simulink model "s_aero2_2dof_lqi"  (R2025a)
settings: Solver=ode4  StartTime=0.0  StopTime=30  FixedStep=0.002  RelTol=1e-3
values from neighbouring files (symbols this model uses):
  A = [0 0 1 0 0 0 ... (first row only)    [aero2_2dof_control_lqi.m]
  B = [0 0; 0 0; 0 0; 0 0; Kpp*Dt/Jp Kpy*Dt/Jp; Kyp*Dt/Jy Kyy*Dt/Jy]    [aero2_2dof_control_lqi.m]
  C = [0 0 1 0 0 0; 0 0 0 1 0 0]    [aero2_2dof_control_lqi.m]
  D = zeros(2)    [aero2_2dof_control_lqi.m]
  K = lqr(A, B, Q, R)    [aero2_2dof_control_lqi.m]
libraries: simulink_extras x4, quarc_library x4
settings Model: Creator=MLevis  LastModifiedBy=khanh
settings DataIOCC: ReturnWorkspaceOutputs=off
settings DebuggingCC: UnconnectedInputMsg=warning  UnconnectedOutputMsg=warning  UnconnectedLineMsg=warning
settings ModelReferenceCC: EnableRefExpFcnMdlSchedulingChecks=on
settings RTWCC: GPUComputeCapability=3.5  DLArmComputeVersion=19.05

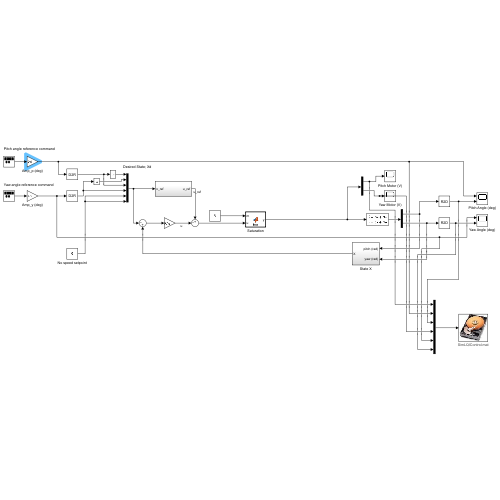
[thumbnail: Simulink's stored preview of the top-level diagram]
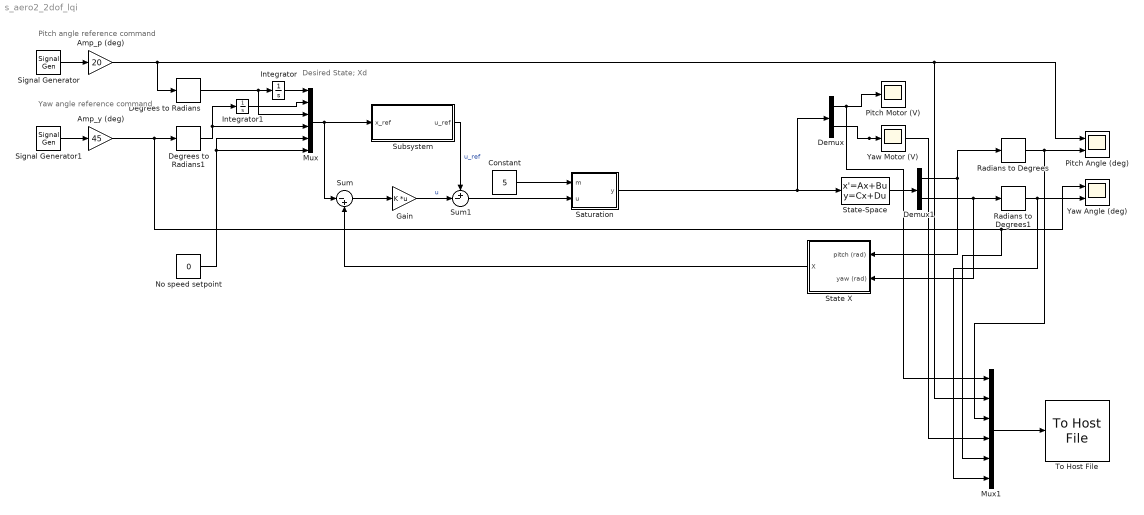
== system s_aero2_2dof_lqi ==
  note: Pitch angle reference command
  note: Desired State; Xd
  note: Yaw angle reference command
  Amp_p (deg) : Gain  Gain=20
  Amp_y (deg) : Gain  Gain=45
  Constant : Constant  Value=5
  Degrees to Radians : simulink_extras/Transformations/Degrees to Radians
  Degrees to Radians1 : simulink_extras/Transformations/Degrees to Radians
  Demux : Demux  Outputs=2
  Demux1 : Demux  Outputs=2
  Gain : Gain  Gain=K  Multiplication=Matrix(K*u)
  Integrator : Integrator
  Integrator1 : Integrator
  Mux : Mux  Inputs=6
  Mux1 : Mux  Inputs=6
  No speed setpoint : Constant  Value=0
  Pitch Angle (deg) : Scope  NumInputPorts=2
      settings: ActiveDisplayYMinimum=-37.565994461674038  ActiveDisplayYMaximum=37.585053253511326  DataLoggingVariableName=Aero2_LQR_Sim_Pitch
  Pitch Motor (V) : Scope
      settings: ActiveDisplayYMinimum=-30.03402684903477  ActiveDisplayYMaximum=30.033448635041648  DataLoggingVariableName=Aero2_LQR_Sim_Vp
  Radians to Degrees : simulink_extras/Transformations/Radians to Degrees
  Radians to Degrees1 : simulink_extras/Transformations/Radians to Degrees
  Saturation : MATLAB Function  TreatAsAtomicUnit=on
  Signal Generator : SignalGenerator  WaveForm=square  Frequency=0.05
  Signal Generator1 : SignalGenerator  WaveForm=square  Frequency=0.04
  State X : Subsystem
  State-Space : StateSpace  A=A  B=B  C=C  D=D  InitialCondition=0
  Subsystem : Subsystem
  Sum : Sum  Inputs=|-+
  Sum1 : Sum  Inputs=+-|
  To Host File : quarc_library/Sinks/To Host/To Host File  source=Specify via dialog (do not evaluate)  file_name=SimLQIControl.mat  variable_name=SimLQIControl  decimation=1  sample_time=-1  file_format=MAT-file v.4  options=No header or footer  append=off  final_file_name=SimLQIControl.mat  encoding=Default  bitrate=2000000
  Yaw Angle (deg) : Scope  NumInputPorts=2
      settings: ActiveDisplayYMinimum=-107.4635266108982  ActiveDisplayYMaximum=107.4641320951424  DataLoggingVariableName=Aero2_LQR_Sim_Yaw
  Yaw Motor (V) : Scope
      settings: ActiveDisplayYMinimum=-30.005517529091861  ActiveDisplayYMaximum=30.005359660360352  DataLoggingVariableName=Aero2_LQR_Sim_Vy
  wires:
  No speed setpoint/1 -> Mux/5, Mux/6
  Sum/1 -> Gain/1
  Demux1/2 -> State X/2(yaw (rad)), Radians to Degrees1/1
  Saturation/1(y) -> Demux/1, State-Space/1
  Signal Generator1/1 -> Amp_y (deg)/1
  Mux/1 -> Subsystem/1(x_ref), Sum/1
  State-Space/1 -> Demux1/1
  Demux1/1 -> State X/1(pitch (rad)), Radians to Degrees/1
  State X/1(X) -> Sum/2
  Gain/1 -> Sum1/2  "u"
  Signal Generator/1 -> Amp_p (deg)/1
  Degrees to Radians/1 -> Mux/3, Integrator/1
  Degrees to Radians1/1 -> Integrator1/1, Mux/4
  Integrator/1 -> Mux/1
  Integrator1/1 -> Mux/2
  Subsystem/1(u_ref) -> Sum1/1  "u_ref"
  Constant/1 -> Saturation/1(m)
  Sum1/1 -> Saturation/2(u)
  Mux1/1 -> To Host File/1
  Radians to Degrees/1 -> Mux1/3, Pitch Angle (deg)/2
  Demux/1 -> Mux1/1, Pitch Motor (V)/1
  Radians to Degrees1/1 -> Mux1/6, Yaw Angle (deg)/2
  Amp_p (deg)/1 -> Mux1/2, Pitch Angle (deg)/1, Degrees to Radians/1
  Amp_y (deg)/1 -> Mux1/5, Yaw Angle (deg)/1, Degrees to Radians1/1
  Demux/2 -> Mux1/4, Yaw Motor (V)/1

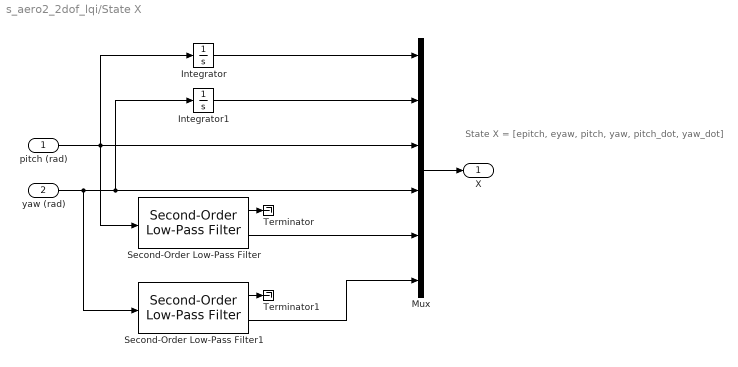
== system s_aero2_2dof_lqi/State X ==
  note: State X = [epitch, eyaw, pitch, yaw, pitch_dot, yaw_dot]
  pitch (rad) : Inport
  yaw (rad) : Inport  Port=2
  Integrator : Integrator
  Integrator1 : Integrator
  Mux : Mux  Inputs=6
  Second-Order Low-Pass Filter : quarc_library/Continuous/Second-Order Low-Pass Filter  params_source=Internal (dialog parameters)  input_width=50  input_zeta=0.8  input_init=0
  Second-Order Low-Pass Filter1 : quarc_library/Continuous/Second-Order Low-Pass Filter  params_source=Internal (dialog parameters)  input_width=50  input_zeta=0.8  input_init=0
  Terminator : Terminator
  Terminator1 : Terminator
  X : Outport
  wires:
  Mux/1 -> X/1
  yaw (rad)/1 -> Integrator1/1, Mux/4, Second-Order Low-Pass Filter1/1
  pitch (rad)/1 -> Second-Order Low-Pass Filter/1, Integrator/1, Mux/3
  Second-Order Low-Pass Filter/2 -> Mux/5
  Second-Order Low-Pass Filter1/2 -> Mux/6
  Second-Order Low-Pass Filter/1 -> Terminator/1
  Second-Order Low-Pass Filter1/1 -> Terminator1/1
  Integrator/1 -> Mux/1
  Integrator1/1 -> Mux/2

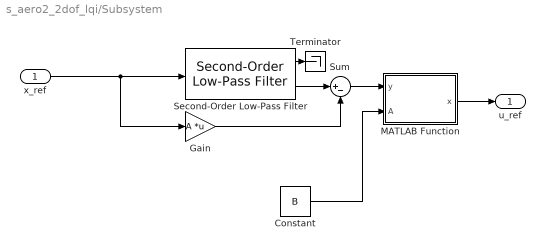
== system s_aero2_2dof_lqi/Subsystem ==
  x_ref : Inport
  Constant : Constant  Value=B
  Gain : Gain  Gain=A  Multiplication=Matrix(K*u)
  MATLAB Function : MATLAB Function  TreatAsAtomicUnit=on
  Second-Order Low-Pass Filter : quarc_library/Continuous/Second-Order Low-Pass Filter  params_source=Internal (dialog parameters)  input_width=50  input_zeta=0.8  input_init=0
  Sum : Sum  Inputs=|+-
  Terminator : Terminator
  u_ref : Outport
  wires:
  x_ref/1 -> Gain/1, Second-Order Low-Pass Filter/1
  Second-Order Low-Pass Filter/1 -> Terminator/1
  Second-Order Low-Pass Filter/2 -> Sum/1
  Gain/1 -> Sum/2
  Sum/1 -> MATLAB Function/1(y)
  Constant/1 -> MATLAB Function/2(A)
  MATLAB Function/1(x) -> u_ref/1

== matlab function s_aero2_2dof_lqi/Subsystem/MATLAB Function ==
  data: y input; x output; A input
function x = u_ref(y, A)

x = A\y

== matlab function s_aero2_2dof_lqi/Saturation ==
  data: m input; u input; y output
function y = fcn(m,u)
    u_min = -24;
    u_max = 24;
y = ((u_min + u_max) + ...
         u_min .* tanh((u_min - u)*m) + ...
         u_max .* tanh((u - u_max)* m) + ...
         u .* (tanh((u - u_min)*m) - tanh((u - u_max)*m)))./2;
